simulink model "nncontroller_5_50"  (R2021a)
settings: Solver=VariableStepAuto  StartTime=0.0  StopTime=10.0  RelTol=1e-3
libraries: neural x257
(part 14 of 14)

== system nncontroller_5_50/Feed-Forward Neural Network/Layer 6/Delays 1 ==
  "p{6}" : Inport  PortDimensions=50
      mask Display: e = 0.06;c1 = [120 230 180]/255;c2 = ([120 230 180]+0)/(256+128);c3 = ([120 230 180]+128)/(256+128);patch([0 1 1 0],[0 0 1 1],c1);patch([0 1 1 1-e 1-e 0+e],[0 0 1 1-e 0+e 0+e],c2);patch([0 0 1 1-e 0+e 0+e],[0 1 1 1-e 1-e 0+e],c3);plot([0 1 1 0 0],[0 0 1 1 0]);
  mux : Mux  Inputs=1
      mask Display: e = 0.06;c1 = [120 150 230]/255;c2 = ([120 150 230]+0)/383;c3 = ([120 150 230]+128)/383;patch([0 1 1 0],[0 0 1 1],c1);patch([0 1 1 1-e 1-e 0+e],[0 0 1 1-e 0+e 0+e],c2);patch([0 0 1 1-e 0+e 0+e],[0 1 1 1-e 1-e 0+e],c3);plot([0 1 1 0 0],[0 0 1 1 0]);disp('Mux')
  "pd{6,5}" : Outport
      mask Display: e = 0.06;c1 = [120 230 180]/255;c2 = ([120 230 180]+0)/(256+128);c3 = ([120 230 180]+128)/(256+128);patch([0 1 1 0],[0 0 1 1],c1);patch([0 1 1 1-e 1-e 0+e],[0 0 1 1-e 0+e 0+e],c2);patch([0 0 1 1-e 0+e 0+e],[0 1 1 1-e 1-e 0+e],c3);plot([0 1 1 0 0],[0 0 1 1 0]);
  wires:
  "p{6}"/1 -> mux/1
  mux/1 -> "pd{6,5}"/1

== system nncontroller_5_50/Feed-Forward Neural Network/Layer 6/LW{6,5} ==
  "ad{6,5}" : Inport  PortDimensions=50
      mask Display: e = 0.06;c1 = [120 230 180]/255;c2 = ([120 230 180]+0)/(256+128);c3 = ([120 230 180]+128)/(256+128);patch([0 1 1 0],[0 0 1 1],c1);patch([0 1 1 1-e 1-e 0+e],[0 0 1 1-e 0+e 0+e],c2);patch([0 0 1 1-e 0+e 0+e],[0 1 1 1-e 1-e 0+e],c3);plot([0 1 1 0 0],[0 0 1 1 0]);
  "IW{6,5}(1,:)'" : Constant  Value=[0.17741968366688276592668671582941897213459014892578125;-0.51840372245058052858013297736761160194873809814453125;-0.9944374074689033005114424668136052787303924560546875;-0.9216468861613404950361427836469374597072601318359375;0.28460413530149963889925857074558734893798828125;0.325830401253256685123460556496866047382354736328125;0.9441094577286184286180059643811546266078948974609375;0.5268168479042556473501690561533905565738677978515625;-0.23174375094860100166016536604729481041431427001953125;0.66972858285246250620303953837719745934009552001953125;0.7468657501883406713005797428195364773273468017578125;-0.26173402184740213183289370135753415524959564208984375;0.9113792024887847897929304963327012956142425537109375;-0.168561040304518960919466508130426518619060516357421875;0.74056630290849856379509219550527632236480712890625;0.926556436576102981916847056709229946136474609375;-0.1411265795596066408013058435244602151215076446533203125;0.27022170849392812552736131692654453217983245849609375;-0.98737826322670374512568969294079579412937164306640625;-0.5746835395186133954581464422517456114292144775390625;-0.1534709884597249551774211795418523252010345458984375;0.68342813531677160110433533191098831593990325927734375;0.91524024156598482448998765903525054454803466796875;-0.77552818144633051122838196533848531544208526611328125;-0.36358346359929327729076931063900701701641082763671875;-0.3798285172899193984363819254213012754917144775390625;0.7785489034314438949735404094099067151546478271484375;-0.592170989197118746716341775027103722095489501953125;0.1700456330609891875127459570649079978466033935546875;-0.1527573549652438134049958762261667288839817047119140625;-0.549276021239939016282960437820293009281158447265625;-0.89757560095102828512381165637634694576263427734375;0.4207216845240377978143442305736243724822998046875;-0.523712682441344501427238355972804129123687744140625;-0.5432622333264560676724386212299577891826629638671875;0.1591739599666414928247348825607332400977611541748046875;-0.976028080095645567126894093235023319721221923828125;0.2058423127048156775487086633802391588687896728515625;0.8877068244884303016561943877604790031909942626953125;-0.98482228141156447076554059094632975757122039794921875;0.388931339986295310229280630665016360580921173095703125;0.494857507312737976423733243791502900421619415283203125;-0.97047359120844955970852652171743102371692657470703125;0.29879048566982080448184433407732285559177398681640625;-0.76925069008126045755346922305761836469173431396484375;-0.383864012497631412745846546386019326746463775634765625;0.200811716008007234979260147156310267746448516845703125;0.254851566450577993183657099507399834692478179931640625;0.5463936196451351090530579313053749501705169677734375;0.78942545389395368804485997316078282892704010009765625]
      mask Display: e = 0.06;c1 = [120 150 230]/255;c2 = ([120 150 230]+0)/383;c3 = ([120 150 230]+128)/383;patch([0 1 1 0],[0 0 1 1],c1);patch([0 1 1 1-e 1-e 0+e],[0 0 1 1-e 0+e 0+e],c2);patch([0 0 1 1-e 0+e 0+e],[0 1 1 1-e 1-e 0+e],c3);plot([0 1 1 0 0],[0 0 1 1 0]);disp('weights');
  Mux : Mux  Inputs=1
      mask Display: e = 0.06;c1 = [120 150 230]/255;c2 = ([120 150 230]+0)/383;c3 = ([120 150 230]+128)/383;patch([0 1 1 0],[0 0 1 1],c1);patch([0 1 1 1-e 1-e 0+e],[0 0 1 1-e 0+e 0+e],c2);patch([0 0 1 1-e 0+e 0+e],[0 1 1 1-e 1-e 0+e],c3);plot([0 1 1 0 0],[0 0 1 1 0]);disp('Mux');
  dotprod1 : neural/Weight Functions/dotprod
  "lz{6,5}" : Outport
      mask Display: e = 0.06;c1 = [120 230 180]/255;c2 = ([120 230 180]+0)/(256+128);c3 = ([120 230 180]+128)/(256+128);patch([0 1 1 0],[0 0 1 1],c1);patch([0 1 1 1-e 1-e 0+e],[0 0 1 1-e 0+e 0+e],c2);patch([0 0 1 1-e 0+e 0+e],[0 1 1 1-e 1-e 0+e],c3);plot([0 1 1 0 0],[0 0 1 1 0]);
  wires:
  "IW{6,5}(1,:)'"/1 -> dotprod1/1
  "ad{6,5}"/1 -> dotprod1/2
  dotprod1/1 -> Mux/1
  Mux/1 -> "lz{6,5}"/1
